simulink model "JONASBROTHERS"  (R2021b)
settings: Solver=FixedStepAuto  StartTime=0.0  StopTime=20  FixedStep=0.0001  RelTol=1e-3
model workspace (MATLAB code in the model file):
  | %% Parameters
  | m_pl = 8800;
  | r_d = 0.2323/2;
  | ig = 4;
  | J_drum = 1.0;
  | J_M = 1.5;
  | %J_M = 2.9;
  | b_hat = 15;
  | 
  | %% Speed Controller
  | t_r = 1e-3;
  | w_BW = log(9)/t_r;
  | %w_BW = 749.6586;
  | w_BWs = 0.1*w_BW;
  | %w_BWs = log(9)/0.09;
  | J_hat = m_pl*((r_d/(ig*4))^2) + J_drum*((1/ig)^2) + J_M
  | 
  | np=2;
  | p=4;
  | i_d_nl = 37.46;
  | %i_d_nl = 65.32;
  | 
  | %% Electrical Parameters
  | R_R_opt = 0.0193;
  | %R_R_opt = 0.04264;
  | R_R_hat = R_R_opt;
  | X_M_opt = 2.81;
  | %X_M_opt = 1.5829;
  | X_sig_opt = 0.0445;
  | %X_sig_opt = 0.0250;
  | omega_rN = 310.5988;
  | omega_N = 314.1593;
  | omega1 = omega_rN;
  | 
  | L_M_hat = X_M_opt/omega1;
  | L_sig_hat = X_sig_opt/omega1;
  | R_s = 0.04264;
  | %R_s = R_R_hat*1.5;
  | %psi_ref = L_M_hat * i_d_nl;
  | psi_ref = 0.8537;
  | %psi_ref = 0.70;
  | KVA = 90/0.85;
  | %V_base = (KVA*1000)/(160*1.73);
  | V_base = 400*sqrt(2)/sqrt(3);
  | alpha_fw = (2*R_R_hat)/L_sig_hat;
  | Ts = 0.0001;
  | I_max = 185;
  | 
  | kps = 2*J_hat*w_BWs/(3*np^2*psi_ref); % notes psi_R_hat is psi_ref
  | kis = w_BWs^2*2*J_hat/(3*np^2*psi_ref); % notes
  | Ba = 2*J_hat/(3*np^2*psi_ref)*(w_BWs-b_hat/J_hat); % notes
  | 
  | kp = w_BW*L_sig_hat;
  | ki = w_BW^2*L_sig_hat;
  | Ra = w_BW*L_sig_hat - (R_R_hat + R_s);
  | R = R_R_hat + R_s;
  | %% Noise
  | sigma_w = 0.5;
  | beta = 10000;
undefined symbols (not defined in the file or in its folder): j, magnitude
libraries: fl_lib x22, nesl_utility x9, CustomComponents_lib x6, simulink x6, slpidlib x2, sdl_lib x1, SignalEditorBlockLib x1
(part 1 of 2)
settings Model: Creator=Jakob  LastModifiedBy=Jakob
settings DebuggingCC: UnconnectedInputMsg=none  UnconnectedOutputMsg=none  UnconnectedLineMsg=none
settings RTWCC: DLArmComputeVersion=20.02.1

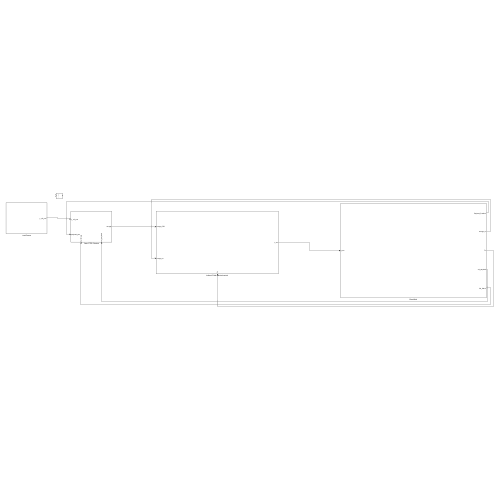
[thumbnail: Simulink's stored preview of the top-level diagram]
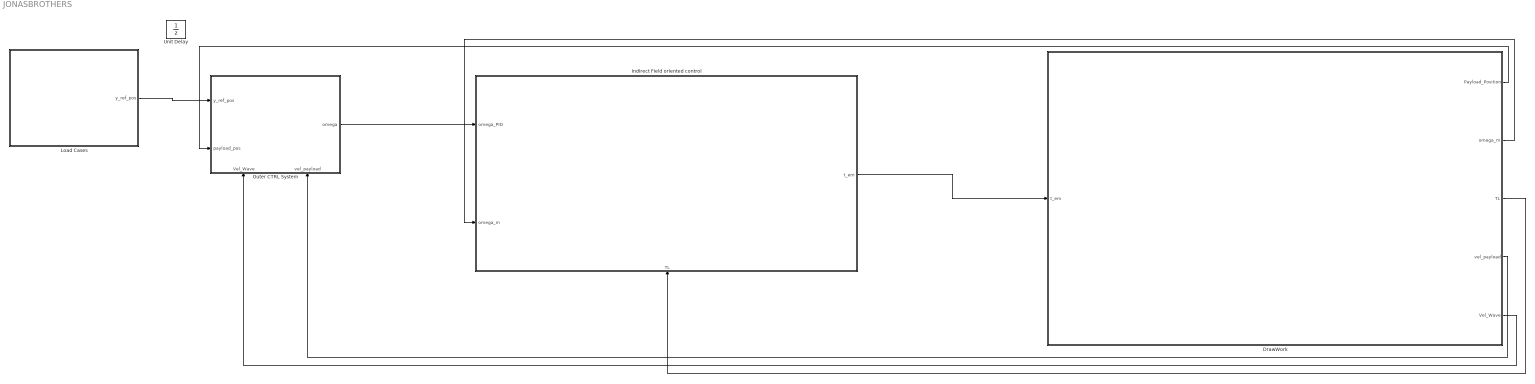
== system JONASBROTHERS ==
  DrawWork : Subsystem
  Indirect Field oriented control : Subsystem
      settings: PortSchema="{\"entries\":[{\"content\":{\"sides\":[{\"content\":{\"connectorIds\":[\"In1\",\"In2\"]},\"type\":\"ConnectorPlacement.EquallySpacedRectSide\",\"uuid\":\"3558566d-3896-4be7-a448-342d07425086\"},{\"content\":{\"connectorIds\":[\"Out1\"],\"side\":\"RIGHT\"},\"type\":\"ConnectorPlacement.EquallySpacedRectSide\",\"uuid\":\"82264b61-0ebe-4d2c-998d-795058aae34e\"},{\"content\":{\"connectorIds\":[],\"side\":\"TOP\"},\"type\":\"ConnectorPlacement.EquallySpacedRectSide\",\"uuid\":\"470bd7e5-a451-470c-b822-89589bfb916a\"},{\"content\":{\"connectorIds\":[\"In3\"],\"side\":\"BOTTOM\"},\"type\":\"ConnectorPlacement.EquallySpacedRectSide\",\"uuid\":\"a5dc14f8-1aa2-4f6b-8a94-10f64ecc4440\"}]},\"type\":\"ConnectorPlacement.EquallySpacedConnector\",\"uuid\":\"fc603cd1-8d61-44a9-91b8-960bbff8932a\"}],\"packageUris\":[\"http://schema.mathworks.com/mf0/Connector/R2020b\"],\"version\":\"1.0\"}"
  Load Cases : Subsystem
  Outer CTRL System : Subsystem
      settings: PortSchema="{\"entries\":[{\"content\":{\"sides\":[{\"content\":{\"connectorIds\":[\"In1\",\"In2\"]},\"type\":\"ConnectorPlacement.EquallySpacedRectSide\",\"uuid\":\"1b9d5986-b048-41c2-8e20-8e14a10e87ac\"},{\"content\":{\"connectorIds\":[\"Out1\"],\"side\":\"RIGHT\"},\"type\":\"ConnectorPlacement.EquallySpacedRectSide\",\"uuid\":\"6d417e58-246f-4168-97e0-db5100f5a916\"},{\"content\":{\"connectorIds\":[],\"side\":\"TOP\"},\"type\":\"ConnectorPlacement.EquallySpacedRectSide\",\"uuid\":\"d5ccf72e-5ab0-4bd7-afc9-f09220873e53\"},{\"content\":{\"connectorIds\":[\"In3\",\"In4\"],\"side\":\"BOTTOM\"},\"type\":\"ConnectorPlacement.EquallySpacedRectSide\",\"uuid\":\"d857e7ff-cab5-40fc-8d38-72d8a9d59103\"}]},\"type\":\"ConnectorPlacement.EquallySpacedConnector\",\"uuid\":\"d6c41efc-b86a-43cb-98a1-4acad2c3d840\"}],\"packageUris\":[\"http://schema.mathworks.com/mf0/Connector/R2020b\"],\"version\":\"1.0\"}"
  Unit Delay : UnitDelay  SampleTime=-1  HasFrameUpgradeWarning=on
  wires:
  DrawWork/1(Payload_Position) -> Outer CTRL System/2(payload_pos)
  DrawWork/2(omega_m) -> Indirect Field oriented control/2(omega_m)
  DrawWork/3(TL) -> Indirect Field oriented control/3(TL)
  Outer CTRL System/1(omega) -> Indirect Field oriented control/1(omega_PID)
  Indirect Field oriented control/1(t_em) -> DrawWork/1(t_em)
  DrawWork/5(Vel_Wave) -> Outer CTRL System/3(Vel_Wave)
  Load Cases/1(y_ref_pos) -> Outer CTRL System/1(y_ref_pos)
  DrawWork/4(vel_payload) -> Outer CTRL System/4(vel_payload)

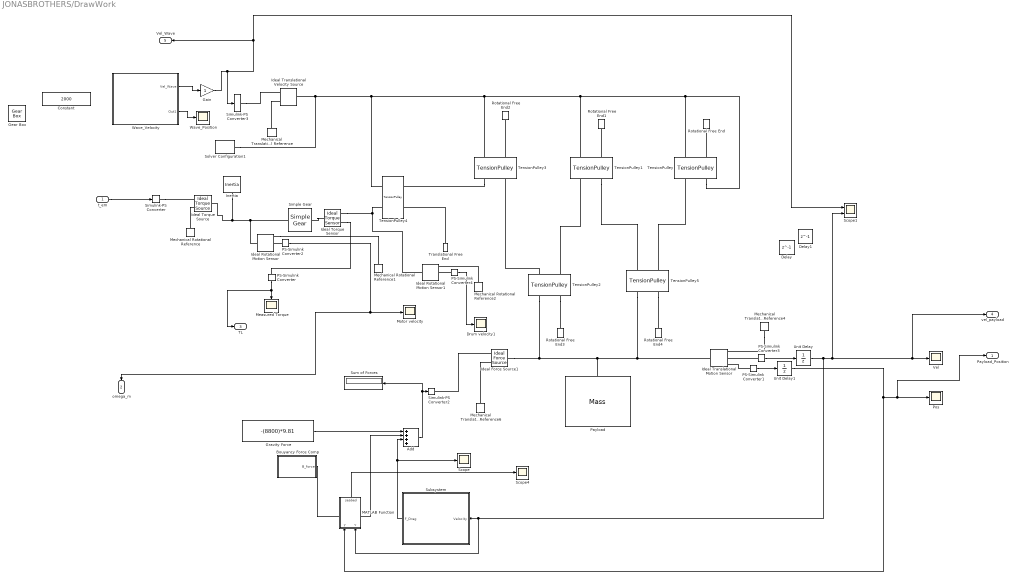
== system JONASBROTHERS/DrawWork ==
  t_em : Inport
  Add : Sum  Inputs=++++
  Bouyancy Force Comp : Subsystem
  Constant : Constant  Value=2000
  Delay : Delay  DelayLength=1  InitialCondition=75
  Delay1 : Delay  DelayLength=1  InitialCondition=0
  Drum velocity1 : Scope
  Gain : Gain
  Gear Box : fl_lib/Mechanical/Mechanisms/Gear Box  ratio=1  t_in_specify=off  t_in_priority=None  t_in=0 N*m  t_in_nominal_specify=off  t_in_nominal_unit=N*m  t_in_nominal_value=1  t_out_specify=off  t_out_priority=None  t_out=0 N*m  t_out_nominal_specify=off  t_out_nominal_unit=N*m  t_out_nominal_value=1
      settings: SourceProductBaseCode=PW,SS,VE
  Gravity Force : Constant  Value=-(8800)*9.81
  Ideal Force Source1 : fl_lib/Mechanical/Mechanical Sources/Ideal Force Source
      settings: SourceProductBaseCode=PW,SS,VE
  Ideal Rotational Motion Sensor : fl_lib/Mechanical/Mechanical Sensors/Ideal Rotational Motion Sensor  wrap_angle=simscape.enum.onoff.off  offset=0 rad
      settings: SourceProductBaseCode=PW,SS,VE
  Ideal Rotational Motion Sensor1 : fl_lib/Mechanical/Mechanical Sensors/Ideal Rotational Motion Sensor  wrap_angle=simscape.enum.onoff.off  offset=0 rad
      settings: SourceProductBaseCode=PW,SS,VE
  Ideal Torque Sensor : fl_lib/Mechanical/Mechanical Sensors/Ideal Torque Sensor
      settings: SourceProductBaseCode=PW,SS,VE
  Ideal Torque Source : fl_lib/Mechanical/Mechanical Sources/Ideal Torque Source
      settings: SourceProductBaseCode=PW,SS,VE
  Ideal Translational Motion Sensor : fl_lib/Mechanical/Mechanical Sensors/Ideal Translational Motion Sensor  offset=75 m
      settings: SourceProductBaseCode=PW,SS,VE
  Ideal Translational Velocity Source : fl_lib/Mechanical/Mechanical Sources/Ideal Translational Velocity Source
      settings: SourceProductBaseCode=PW,SS,VE
  Inertia : fl_lib/Mechanical/Rotational Elements/Inertia  inertia=1.5 kg*m^2  num_ports=foundation.enum.numPorts2.one  w_specify=off  w_priority=High  w=0 rad/s  w_nominal_specify=off  w_nominal_unit=rad/s  w_nominal_value=1  t_specify=off  t_priority=None  t=0 N*m  t_nominal_specify=off  t_nominal_unit=N*m  t_nominal_value=1
      settings: SourceProductBaseCode=PW,SS,VE
  MATLAB Function : MATLAB Function  TreatAsAtomicUnit=on
  Measured Torque : Scope
  Mechanical Rotational Reference : fl_lib/Mechanical/Rotational Elements/Mechanical Rotational Reference
      settings: SourceProductBaseCode=PW,SS,VE
  Mechanical Rotational Reference1 : fl_lib/Mechanical/Rotational Elements/Mechanical Rotational Reference
      settings: SourceProductBaseCode=PW,SS,VE
  Mechanical Rotational Reference2 : fl_lib/Mechanical/Rotational Elements/Mechanical Rotational Reference
      settings: SourceProductBaseCode=PW,SS,VE
  Mechanical Translational Reference : fl_lib/Mechanical/Translational Elements/Mechanical Translational Reference
      settings: SourceProductBaseCode=PW,SS,VE
  Mechanical Translational Reference4 : fl_lib/Mechanical/Translational Elements/Mechanical Translational Reference
      settings: SourceProductBaseCode=PW,SS,VE
  Mechanical Translational Reference6 : fl_lib/Mechanical/Translational Elements/Mechanical Translational Reference
      settings: SourceProductBaseCode=PW,SS,VE
  Motor velocity : Scope
  PS-Simulink Converter{,1..4} (5 alike) : nesl_utility/PS-Simulink Converter  PhysicalDomain=network_engine_domain  SubClassName=ps_output  LeftPortType=input  RightPortType=output  PseudoPeriodic=off  Frequencies=[]  VectorFormat=inherit  Unit=inherit  AffineConversion=off
      settings: SourceProductBaseCode=SS,PW,VE
  Payload : fl_lib/Mechanical/Translational Elements/Mass  mass=8800 kg  num_ports=foundation.enum.numPorts2.one  v_specify=off  v_priority=High  v=0 m/s  v_nominal_specify=off  v_nominal_unit=m/s  v_nominal_value=1  f_specify=off  f_priority=None  f=0 N  f_nominal_specify=off  f_nominal_unit=N  f_nominal_value=1
      settings: SourceProductBaseCode=PW,SS,VE
  Pos : Scope
  Rotational Free End{,1..4} (5 alike) : fl_lib/Mechanical/Rotational Elements/Rotational Free End  w_specify=off  w_priority=None  w=0 rad/s  w_nominal_specify=off  w_nominal_unit=rad/s  w_nominal_value=1
      settings: SourceProductBaseCode=PW,SS,VE
  Scope : Scope
  Scope1 : Scope  NumInputPorts=2
  Scope4 : Scope
  Simple Gear : sdl_lib/Gears/Simple Gear  ratio=4  rotation_direction=sdl.enum.shaftOutputDirection.same  friction_model=sdl.enum.gear_efficiencies_load.off  T_noload=0.1 N*m  T_nom=5 N*m  efficiency_nom=0.8  efficiency=0.8  temperature_TLU=[280, 300, 320] K  load_TLU=[1, 5, 10] N*m  efficiency_TLU=[.95, .9, .85]  efficiency_TLU2=[.85, .8, .75; .95, .9, .85; .85, .8, .7]  w_thr=0.01 rad/s  pwr_thr=0.001 W  backlash_model=sdl.enum.backlashModel.Off  backlash_distance=1e-3 mm  x0=0 mm  r_base=0.1 m  hardstop_model=simscape.enum.hardstop.smooth  transition=1e-4 mm  backlash_stiffness=1e7 N/m  backlash_damping=1e6 N*s/m  e=0  v_tol=0.001 m/s  mu_visc=[0, 0] N*m*s/rad  enable_faults=simscape.enum.onoff.off  efficiency_fault=0.05  external_fault=simscape.enum.onoff.off  temporal_fault=simscape.enum.onoff.off  fault_time=5 s  fault_angles=pi / 12 rad  report_fault=simscape.enum.assert.action.none  thermal_mass=50 J/K  temperature_specify=off  temperature_priority=High  temperature=300 K  temperature_nominal_specify=off  temperature_nominal_unit=K  temperature_nominal_value=1  x_backlash_specify=off  x_backlash_priority=None  x_backlash=0 mm  x_backlash_nominal_specify=off  x_backlash_nominal_unit=mm  x_backlash_nominal_value=1  f_hardstop_specify=off  f_hardstop_priority=None  f_hardstop=0 N  f_hardstop_nominal_specify=off  f_hardstop_nominal_unit=N  f_hardstop_nominal_value=1  v_backlash_specify=off  v_backlash_priority=None  v_backlash=0 m/s  v_backlash_nominal_specify=off  v_backlash_nominal_unit=m/s  v_backlash_nominal_value=1
  Simulink-PS Converter : nesl_utility/Simulink-PS Converter  PhysicalDomain=network_engine_domain  SubClassName=ps_input  LeftPortType=input  RightPortType=output  PseudoPeriodic=off  Frequencies=[]  NoiseDistribution=none  NoiseParameters=[]  Unit=N*m  AffineConversion=off  FilteringAndDerivatives=provide  SimscapeFilterOrder=1  InputFilterTimeConstant=0.001  UdotUserProvided=0
      settings: SourceProductBaseCode=SS,PW,VE
  Simulink-PS Converter2 : nesl_utility/Simulink-PS Converter  PhysicalDomain=network_engine_domain  SubClassName=ps_input  LeftPortType=input  RightPortType=output  PseudoPeriodic=off  Frequencies=[]  NoiseDistribution=none  NoiseParameters=[]  Unit=N  AffineConversion=off  FilteringAndDerivatives=provide  SimscapeFilterOrder=1  InputFilterTimeConstant=0.001  UdotUserProvided=0
      settings: SourceProductBaseCode=SS,PW,VE
  Simulink-PS Converter3 : nesl_utility/Simulink-PS Converter  PhysicalDomain=network_engine_domain  SubClassName=ps_input  LeftPortType=input  RightPortType=output  PseudoPeriodic=off  Frequencies=[]  NoiseDistribution=none  NoiseParameters=[]  Unit=m/s  AffineConversion=off  FilteringAndDerivatives=filter  SimscapeFilterOrder=1  InputFilterTimeConstant=0.001  UdotUserProvided=0
      settings: SourceProductBaseCode=SS,PW,VE
  Solver Configuration1 : nesl_utility/Solver Configuration  PhysicalDomain=network_engine_domain  SubClassName=solver  LeftPortType=input  RightPortType=generic  Tones=[]  Harmonics=[]  SimulateNoise=off  Profile=off  UseLocalSampling=off  EnableSwitchedLinearOptims=on  FrequencyDomain=off  UseCCode=off  RelTol=0.001  AbsTol=0.001  MinStep=1e-09  ToWorkspace=off  RevertToSquareIcSolve=off  NumHomotopyIterations=100  PhasorMode=off  PhasorModeNumHarmonics=1  IndexReductionMethod=DerivativeReplacement  DoDC=off  ResidualTolerance=1e-06  UseLocalSolver=off  LocalSolverChoice=NE_BACKWARD_EULER_ADVANCER  LocalSolverSampleTime=0.001  DoFixedCost=off  MaxNonlinIter=3  MaxModeIter=2  ComputeImpulses=off  ImpulseIterations=2  LinearAlgebra=auto  LinearAlgebraNumThread=0  EquationFormulation=NE_TIME_EF  DelaysMemoryBudget=1024  AutomaticFiltering=on  FilteringTimeConstant=0.001  PartitionStorageMethod=AS_NEEDED  PartitionMemoryBudget=1024  PartitionMethod=ROBUST
      settings: SourceProductBaseCode=SS,PW,VE
  Subsystem : Subsystem
  Sum of Forces : Display
  TensionPulley{,1..3,5} (5 alike) : CustomComponents_lib/TensionPulley  radius=0.01 m  b_damp=0 N*m*s/rad  inertia=0.001 kg*m^2  mass=0.1 kg  mu_s=1  f_A_specify=off  f_A_priority=None  f_A=0 N  f_A_nominal_specify=off  f_A_nominal_unit=N  f_A_nominal_value=1  f_B_specify=off  f_B_priority=None  f_B=0 N  f_B_nominal_specify=off  f_B_nominal_unit=N  f_B_nominal_value=1  f_C_specify=off  f_C_priority=None  f_C=0 N  f_C_nominal_specify=off  f_C_nominal_unit=N  f_C_nominal_value=1  tau_specify=off  tau_priority=None  tau=0 N*m  tau_nominal_specify=off  tau_nominal_unit=N*m  tau_nominal_value=1  w_specify=off  w_priority=None  w=0 rad/s  w_nominal_specify=off  w_nominal_unit=rad/s  w_nominal_value=1  v_specify=off  v_priority=None  v=0 m/s  v_nominal_specify=off  v_nominal_unit=m/s  v_nominal_value=1
      settings: InternalSimscapePortConfiguration="{\"Bottom\":[],\"Left\":[{\"id\":\"C\",\"label\":\"C\",\"type\":\"foundation.mechanical.translational.translational\"},{\"id\":\"S\",\"label\":\"S\",\"type\":\"foundation.mechanical.rotational.rotational\"}],\"Right\":[{\"id\":\"A\",\"label\":\"A\",\"type\":\"foundation.mechanical.translational.translational\"},{\"id\":\"B\",\"label\":\"B\",\"type\":\"foundation.mechanical.translational.translational\"}],\"Top\":[]}"
  TensionPulley4 : CustomComponents_lib/TensionPulley  radius=0.2323/2 m  b_damp=0.001 N*m*s/rad  inertia=1 kg*m^2  mass=1 kg  mu_s=1  f_A_specify=off  f_A_priority=None  f_A=0 N  f_A_nominal_specify=off  f_A_nominal_unit=N  f_A_nominal_value=1  f_B_specify=off  f_B_priority=None  f_B=0 N  f_B_nominal_specify=off  f_B_nominal_unit=N  f_B_nominal_value=1  f_C_specify=off  f_C_priority=None  f_C=0 N  f_C_nominal_specify=off  f_C_nominal_unit=N  f_C_nominal_value=1  tau_specify=off  tau_priority=None  tau=2000 N*m  tau_nominal_specify=off  tau_nominal_unit=N*m  tau_nominal_value=1  w_specify=off  w_priority=High  w=0 rad/s  w_nominal_specify=off  w_nominal_unit=rad/s  w_nominal_value=1  v_specify=off  v_priority=None  v=0 m/s  v_nominal_specify=off  v_nominal_unit=m/s  v_nominal_value=1
      settings: InternalSimscapePortConfiguration="{\"Bottom\":[],\"Left\":[{\"id\":\"C\",\"label\":\"C\",\"type\":\"foundation.mechanical.translational.translational\"},{\"id\":\"S\",\"label\":\"S\",\"type\":\"foundation.mechanical.rotational.rotational\"}],\"Right\":[{\"id\":\"A\",\"label\":\"A\",\"type\":\"foundation.mechanical.translational.translational\"},{\"id\":\"B\",\"label\":\"B\",\"type\":\"foundation.mechanical.translational.translational\"}],\"Top\":[]}"
  Translational Free End : fl_lib/Mechanical/Translational Elements/Translational Free End  v_specify=off  v_priority=None  v=0 m/s  v_nominal_specify=off  v_nominal_unit=m/s  v_nominal_value=1
      settings: SourceProductBaseCode=PW,SS,VE  InternalSimscapePortConfiguration="{\"Bottom\":[],\"Left\":[{\"id\":\"V\",\"label\":\"\",\"type\":\"foundation.mechanical.translational.translational\"}],\"Right\":[],\"Top\":[]}"
  Unit Delay : UnitDelay  SampleTime=-1  HasFrameUpgradeWarning=on
  Unit Delay1 : UnitDelay  InitialCondition=75  SampleTime=-1  HasFrameUpgradeWarning=on
  Vel : Scope
  Wave_Position : Scope
  Wave_Velocity : Subsystem
  Payload_Position : Outport
  omega_m : Outport  Port=2
  TL : Outport  Port=3
  vel_payload : Outport  Port=4
  Vel_Wave : Outport  Port=5
  wires:
  Subsystem/1(F_Drag) -> Scope/1, Add/3
  Bouyancy Force Comp/1(B_force) -> Add/2
  Wave_Velocity/1(Vel_Wave) -> Gain/1
  Gravity Force/1 -> Add/1
  Add/1 -> Sum of Forces/1, Simulink-PS Converter2/1
  PS-Simulink Converter/1 -> TL/1, Measured Torque/1
  MATLAB Function/1(seabed) -> Scope4/1
  PS-Simulink Converter3/1 -> Unit Delay/1
  PS-Simulink Converter1/1 -> Unit Delay1/1
  Unit Delay/1 -> MATLAB Function/2(v), Subsystem/1(Velocity), vel_payload/1, Vel/1, Scope1/2
  Unit Delay1/1 -> Pos/1, Payload_Position/1, MATLAB Function/1(y)
  t_em/1 -> Simulink-PS Converter/1
  Wave_Velocity/2(Out1) -> Wave_Position/1
  Gain/1 -> Scope1/1, Vel_Wave/1, Simulink-PS Converter3/1
  PS-Simulink Converter4/1 -> Drum velocity1/1
  PS-Simulink Converter2/1 -> Motor velocity/1, omega_m/1
  connections:
  Ideal Force Source1/LConn1 -- TensionPulley2/LConn1 -- TensionPulley5/LConn1 -- Ideal Translational Motion Sensor/LConn1 -- Payload/LConn1
  Simulink-PS Converter/RConn1 -- Ideal Torque Source/RConn1
  Ideal Force Source1/RConn1 -- Simulink-PS Converter2/RConn1
  TensionPulley/LConn2 -- Rotational Free End/LConn1
  Simulink-PS Converter3/RConn1 -- Ideal Translational Velocity Source/RConn1
  PS-Simulink Converter1/LConn1 -- Ideal Translational Motion Sensor/RConn3
  Mechanical Rotational Reference/LConn1 -- Ideal Torque Source/RConn2
  Ideal Force Source1/RConn2 -- Mechanical Translational Reference6/LConn1
  TensionPulley5/LConn2 -- Rotational Free End4/LConn1
  PS-Simulink Converter3/LConn1 -- Ideal Translational Motion Sensor/RConn2
  Mechanical Translational Reference4/LConn1 -- Ideal Translational Motion Sensor/RConn1
  TensionPulley1/LConn2 -- Rotational Free End1/LConn1
  TensionPulley3/LConn2 -- Rotational Free End2/LConn1
  TensionPulley2/LConn2 -- Rotational Free End3/LConn1
  TensionPulley/RConn2 -- TensionPulley4/LConn1 -- Solver Configuration1/RConn1 -- Ideal Translational Velocity Source/LConn1 -- TensionPulley3/LConn1 -- TensionPulley1/LConn1 -- TensionPulley/LConn1
  TensionPulley2/RConn1 -- TensionPulley3/RConn2
  TensionPulley2/RConn2 -- TensionPulley1/RConn1
  TensionPulley1/RConn2 -- TensionPulley5/RConn1
  TensionPulley5/RConn2 -- TensionPulley/RConn1
  Ideal Rotational Motion Sensor/RConn1 -- Mechanical Rotational Reference1/LConn1
  PS-Simulink Converter2/LConn1 -- Ideal Rotational Motion Sensor/RConn2
  Inertia/LConn1 -- Ideal Torque Source/LConn1 -- Ideal Rotational Motion Sensor/LConn1 -- Simple Gear/LConn1
  Ideal Torque Sensor/LConn1 -- Simple Gear/RConn1
  Ideal Torque Sensor/RConn1 -- TensionPulley4/LConn2 -- Ideal Rotational Motion Sensor1/LConn1
  Ideal Torque Sensor/RConn2 -- PS-Simulink Converter/LConn1
  Mechanical Rotational Reference2/LConn1 -- Ideal Rotational Motion Sensor1/RConn1
  PS-Simulink Converter4/LConn1 -- Ideal Rotational Motion Sensor1/RConn2
  Translational Free End/LConn1 -- TensionPulley4/RConn2
  TensionPulley3/RConn1 -- TensionPulley4/RConn1
  Ideal Translational Velocity Source/RConn2 -- Mechanical Translational Reference/LConn1

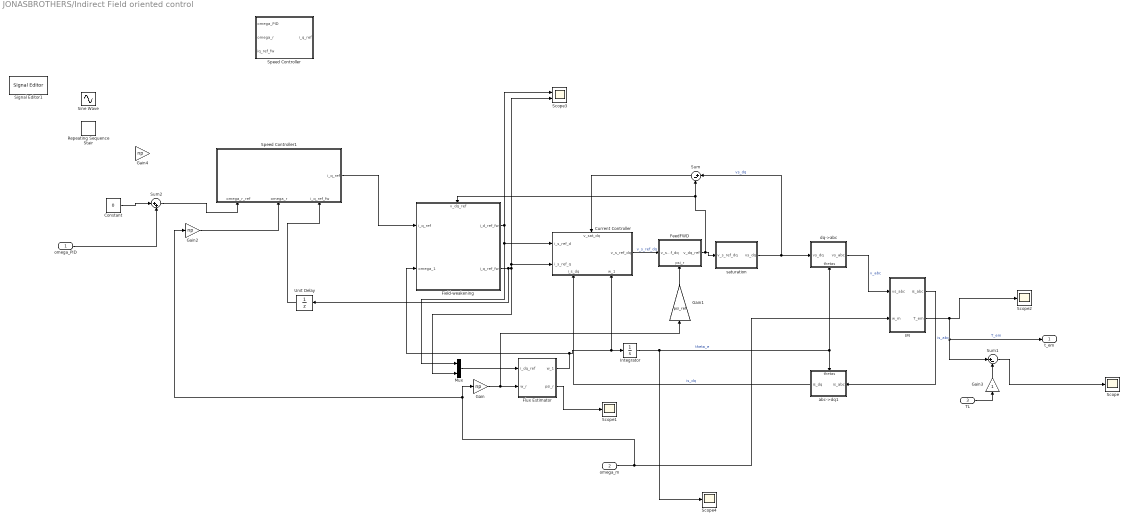
== system JONASBROTHERS/Indirect Field oriented control ==
  omega_PID : Inport
  omega_m : Inport  Port=2
  TL : Inport  Port=3
  Constant : Constant  Value=0
  Current Controller : Subsystem
      settings: PortSchema="{\"entries\":[{\"content\":{\"sides\":[{\"content\":{\"connectorIds\":[\"In1\",\"In2\"]},\"type\":\"ConnectorPlacement.EquallySpacedRectSide\",\"uuid\":\"97c548b6-6990-4323-a853-1e64e742285c\"},{\"content\":{\"connectorIds\":[\"Out1\"],\"side\":\"RIGHT\"},\"type\":\"ConnectorPlacement.EquallySpacedRectSide\",\"uuid\":\"cacb7644-0a67-4de4-9bb2-887734fe331a\"},{\"content\":{\"connectorIds\":[\"In3\"],\"side\":\"TOP\"},\"type\":\"ConnectorPlacement.EquallySpacedRectSide\",\"uuid\":\"a20c1423-7334-426c-a525-8bdb26886bc3\"},{\"content\":{\"connectorIds\":[\"In4\",\"In5\"],\"side\":\"BOTTOM\"},\"type\":\"ConnectorPlacement.EquallySpacedRectSide\",\"uuid\":\"b9821709-22a3-4c1b-ad46-11760bdb190f\"}]},\"type\":\"ConnectorPlacement.EquallySpacedConnector\",\"uuid\":\"74caaff1-86aa-4f34-8e3a-31d84a5552f1\"}],\"packageUris\":[\"http://schema.mathworks.com/mf0/Connector/R2020b\"],\"version\":\"1.0\"}"
  FeedFWD : Subsystem
      settings: AttributesFormatString=%<MinAlgLoopOccurrences>  PortSchema="{\"entries\":[{\"content\":{\"sides\":[{\"content\":{\"connectorIds\":[\"In1\"]},\"type\":\"ConnectorPlacement.EquallySpacedRectSide\",\"uuid\":\"8794a64f-49ba-4da5-9b58-fd7208420cfd\"},{\"content\":{\"connectorIds\":[\"Out1\"],\"side\":\"RIGHT\"},\"type\":\"ConnectorPlacement.EquallySpacedRectSide\",\"uuid\":\"2b8697f1-b735-400e-94f4-d8410b9cec93\"},{\"content\":{\"connectorIds\":[],\"side\":\"TOP\"},\"type\":\"ConnectorPlacement.EquallySpacedRectSide\",\"uuid\":\"d1696b87-b3df-486e-a2ce-05a5a02f4278\"},{\"content\":{\"connectorIds\":[\"In2\"],\"side\":\"BOTTOM\"},\"type\":\"ConnectorPlacement.EquallySpacedRectSide\",\"uuid\":\"350d8cbe-49a8-4b9b-a838-c09ef3fad5b2\"}]},\"type\":\"ConnectorPlacement.EquallySpacedConnector\",\"uuid\":\"fc4af688-7e97-4ab2-a125-9e3e68c4a913\"}],\"packageUris\":[\"http://schema.mathworks.com/mf0/Connector/R2020b\"],\"version\":\"1.0\"}"
  "Field-weakening " : Subsystem
      settings: PortSchema="{\"entries\":[{\"content\":{\"sides\":[{\"content\":{\"connectorIds\":[\"In1\",\"In2\"]},\"type\":\"ConnectorPlacement.EquallySpacedRectSide\",\"uuid\":\"aee381d7-3a71-45d0-966d-7af6601206c5\"},{\"content\":{\"connectorIds\":[\"Out1\",\"Out2\"],\"side\":\"RIGHT\"},\"type\":\"ConnectorPlacement.EquallySpacedRectSide\",\"uuid\":\"b4f04b7a-b16d-4ae2-8d18-1ccf45d54418\"},{\"content\":{\"connectorIds\":[\"In3\"],\"side\":\"TOP\"},\"type\":\"ConnectorPlacement.EquallySpacedRectSide\",\"uuid\":\"7d29b16c-0908-4291-9b7c-a89871d4912d\"}]},\"type\":\"ConnectorPlacement.EquallySpacedConnector\",\"uuid\":\"28c927f9-c9f1-4063-8a99-a2da52e20e9b\"}],\"packageUris\":[\"http://schema.mathworks.com/mf0/Connector/R2020b\"],\"version\":\"1.0\"}"
  Flux Estimator : Subsystem
  Gain : Gain  Gain=np
  Gain1 : Gain  Gain=psi_ref
  Gain2 : Gain  Gain=np
  Gain3 : Gain
  Gain4 : Gain  Gain=np
  IM : Subsystem  mask{R_s=R_s, L_sig=L_sig_hat, R_R=R_R_hat, n_p=2, L_M=L_M_hat}
      mask prompts: R_s "Stator resistance Rs (ohm)"; L_sig "Total leakage inductance L_sig (H)"; R_R "Rotor resistance R_R ( Ohm)"; n_p "Number of pole pairs n_p"; L_M "Magnetising inductance L_M (H)"
      mask help: dynamic model of IM
  Integrator : Integrator
  Mux : Mux  Inputs=2
  Repeating Sequence Stair : simulink/Sources/Repeating Sequence Stair  OutValues=[100 20 30 20 100 50 10 20].'  tsamp=-1  OutMin=[]  OutMax=[]  OutDataTypeStr=double  OutputDataTypeScalingMode=double  OutDataType=fixdt(0,8)  ConRadixGroup=Best Precision: Vector-wise  OutScaling=2^-12
  Scope{,1..2,4} (4 alike) : Scope
  Scope3 : Scope  NumInputPorts=2
  Signal Editor1 : SignalEditorBlockLib/Signal Editor  FileName=input.mat  ActiveScenario=Scenario  ActiveSignal=Signal  IsBus=off  OutputBusObjectStr=Bus: BusObject  SampleTime=0  Interpolate=off  ZeroCross=off  OutputAfterFinalValue=Setting to zero  Unit=inherit  PreserveSignalName=on
  Sine Wave : Sin  Amplitude=150  Frequency=0.5  SampleTime=0
  Speed Controller : Subsystem
  Speed Controller1 : Subsystem
      settings: PortSchema="{\"entries\":[{\"content\":{\"sides\":[{\"content\":{\"connectorIds\":[]},\"type\":\"ConnectorPlacement.EquallySpacedRectSide\",\"uuid\":\"97c548b6-6990-4323-a853-1e64e742285c\"},{\"content\":{\"connectorIds\":[\"Out1\"],\"side\":\"RIGHT\"},\"type\":\"ConnectorPlacement.EquallySpacedRectSide\",\"uuid\":\"cacb7644-0a67-4de4-9bb2-887734fe331a\"},{\"content\":{\"connectorIds\":[],\"side\":\"TOP\"},\"type\":\"ConnectorPlacement.EquallySpacedRectSide\",\"uuid\":\"a20c1423-7334-426c-a525-8bdb26886bc3\"},{\"content\":{\"connectorIds\":[\"In1\",\"In2\",\"In3\"],\"side\":\"BOTTOM\"},\"type\":\"ConnectorPlacement.EquallySpacedRectSide\",\"uuid\":\"b9821709-22a3-4c1b-ad46-11760bdb190f\"}]},\"type\":\"ConnectorPlacement.EquallySpacedConnector\",\"uuid\":\"74caaff1-86aa-4f34-8e3a-31d84a5552f1\"}],\"packageUris\":[\"http://schema.mathworks.com/mf0/Connector/R2020b\"],\"version\":\"1.0\"}"
  Sum : Sum  Inputs=|+-
  Sum1 : Sum  Inputs=|+-
  Sum2 : Sum  Inputs=|++
  Unit Delay : UnitDelay  InitialCondition=160*1.5  SampleTime=-1  HasFrameUpgradeWarning=on
  abc->dq1 : Subsystem
      settings: PortSchema="{\"entries\":[{\"content\":{\"sides\":[{\"content\":{\"connectorIds\":[\"In1\"]},\"type\":\"ConnectorPlacement.EquallySpacedRectSide\",\"uuid\":\"c3863cce-4a98-427c-9e63-89298f679a84\"},{\"content\":{\"connectorIds\":[\"Out1\"],\"side\":\"RIGHT\"},\"type\":\"ConnectorPlacement.EquallySpacedRectSide\",\"uuid\":\"ae3c4991-ab62-4114-9bee-e9a7348a29ce\"},{\"content\":{\"connectorIds\":[\"In2\"],\"side\":\"TOP\"},\"type\":\"ConnectorPlacement.EquallySpacedRectSide\",\"uuid\":\"fea582b6-68e0-450b-8231-0f2cf258215e\"},{\"content\":{\"connectorIds\":[],\"side\":\"BOTTOM\"},\"type\":\"ConnectorPlacement.EquallySpacedRectSide\",\"uuid\":\"4cb5cb50-d1c5-41cc-b580-d3f7a61a133b\"}]},\"type\":\"ConnectorPlacement.EquallySpacedConnector\",\"uuid\":\"936995e1-3667-4d5a-83ac-5ed23eb7cec5\"}],\"packageUris\":[\"http://schema.mathworks.com/mf0/Connector/R2020b\"],\"version\":\"1.0\"}"
  dq->abc : Subsystem
      settings: PortSchema="{\"entries\":[{\"content\":{\"sides\":[{\"content\":{\"connectorIds\":[\"In1\"]},\"type\":\"ConnectorPlacement.EquallySpacedRectSide\",\"uuid\":\"c3863cce-4a98-427c-9e63-89298f679a84\"},{\"content\":{\"connectorIds\":[\"Out1\"],\"side\":\"RIGHT\"},\"type\":\"ConnectorPlacement.EquallySpacedRectSide\",\"uuid\":\"ae3c4991-ab62-4114-9bee-e9a7348a29ce\"},{\"content\":{\"connectorIds\":[],\"side\":\"TOP\"},\"type\":\"ConnectorPlacement.EquallySpacedRectSide\",\"uuid\":\"fea582b6-68e0-450b-8231-0f2cf258215e\"},{\"content\":{\"connectorIds\":[\"In2\"],\"side\":\"BOTTOM\"},\"type\":\"ConnectorPlacement.EquallySpacedRectSide\",\"uuid\":\"09df17c4-38be-4fcd-b44b-abaf9d5b2651\"}]},\"type\":\"ConnectorPlacement.EquallySpacedConnector\",\"uuid\":\"936995e1-3667-4d5a-83ac-5ed23eb7cec5\"}],\"packageUris\":[\"http://schema.mathworks.com/mf0/Connector/R2020b\"],\"version\":\"1.0\"}"
  saturation : Subsystem
  t_em : Outport
  wires:
  Flux Estimator/1(w_1) -> Integrator/1, Current Controller/5(w_1), "Field-weakening "/2(omega_1)
  saturation/1(vs_dq) -> Sum/1, dq->abc/1(vs_dq)  "vs_dq"
  Integrator/1 -> Scope4/1, dq->abc/2(thetas), abc->dq1/2(thetas)  "theta_e"
  dq->abc/1(vs_abc) -> IM/1(vs_abc)  "v_abc"
  IM/1(is_abc) -> abc->dq1/1(is_abc)  "is_abc"
  Flux Estimator/2(psi_r) -> Scope1/1
  Sum/1 -> Current Controller/3(v_sat_dq)
  "Field-weakening "/1(i_d_ref_fw) -> Mux/1, Current Controller/1(i_s_ref_d), Scope3/1
  abc->dq1/1(is_dq) -> Current Controller/4(i_s_dq)  "is_dq"
  Gain/1 -> Gain1/1, Flux Estimator/2(w_r)
  IM/2(T_em) -> t_em/1, Sum1/1, Scope2/1  "T_em"
  Mux/1 -> Flux Estimator/1(i_dq_ref)
  TL/1 -> Gain3/1
  Gain3/1 -> Sum1/2
  "Field-weakening "/2(i_q_ref_fw) -> Unit Delay/1, Scope3/2, Current Controller/2(i_s_ref_q), Mux/2
  Sum1/1 -> Scope/1
  Gain1/1 -> FeedFWD/2(psi_r)
  Current Controller/1(v_s_ref_dq) -> FeedFWD/1(v_s_ref_dq)  "v_s_ref_dq"
  FeedFWD/1(v_dq_ref) -> "Field-weakening "/3(v_dq_ref), Sum/2, saturation/1(v_s_ref_dq)
  Gain2/1 -> Speed Controller1/2(omega_r)
  omega_m/1 -> Gain2/1, Gain/1, IM/2(w_m)
  Unit Delay/1 -> Speed Controller1/3(i_q_ref_fw)
  Constant/1 -> Sum2/1
  Sum2/1 -> Speed Controller1/1(omega_r_ref)
  omega_PID/1 -> Sum2/2
  Speed Controller1/1(i_q_ref) -> "Field-weakening "/1(i_q_ref)

== system JONASBROTHERS/Load Cases ==
  Case Selector : MATLAB Function  TreatAsAtomicUnit=on
  Constant : Constant
  Ramp : simulink/Sources/Ramp  slope=-2.5  start=0  InitialOutput=75
  Ramp1 : simulink/Sources/Ramp  slope=-1  start=0  InitialOutput=15
  Saturation : Saturate  UpperLimit=75  LowerLimit=15
  Saturation1 : Saturate  UpperLimit=15  LowerLimit=0
  Scope : Scope
  y_ref : Constant  Value=75
  y_ref_pos : Outport
  wires:
  Constant/1 -> Case Selector/4(CaseSelector)
  y_ref/1 -> Case Selector/1(Case1)
  Ramp/1 -> Saturation/1
  Saturation/1 -> Case Selector/2(Case2)
  Ramp1/1 -> Saturation1/1
  Saturation1/1 -> Case Selector/3(Case3)
  Case Selector/1(payload_ref_pos) -> Scope/1, y_ref_pos/1

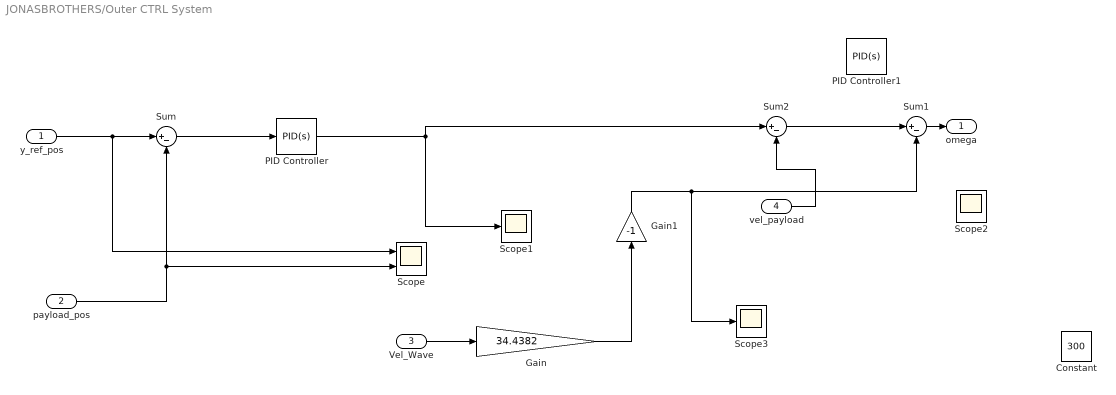
== system JONASBROTHERS/Outer CTRL System ==
  y_ref_pos : Inport
  payload_pos : Inport  Port=2
  Vel_Wave : Inport  Port=3
  vel_payload : Inport  Port=4
  Constant : Constant  Value=300
  Gain : Gain  Gain=34.4382
  Gain1 : Gain  Gain=-1
  PID Controller : slpidlib/PID Controller  Controller=PID  Form=Parallel  TimeDomain=Continuous-time  UseExternalTs=off  SampleTime=-1  IntegratorMethod=Forward Euler  FilterMethod=Forward Euler  ControllerParametersSource=internal  P=20  I=10  D=0  N=100  UseFilter=on  TunerSelectOption=Transfer Function Based (PID Tuner App)  InitialConditionSource=internal  InitialConditionForIntegrator=0  InitialConditionForFilter=0  DifferentiatorICPrevScaledInput=0  ExternalReset=none  TrackingMode=off  Kt=1  LimitOutput=off  SatLimitsSource=internal  UpperSaturationLimit=inf  LowerSaturationLimit=-inf  LinearizeAsGain=on  AntiWindupMode=none  Kb=1  POutMin=[]  POutMax=[]  IOutMin=[]  IOutMax=[]  DOutMin=[]  DOutMax=[]  NOutMin=[]  NOutMax=[]  SumOutMin=[]  SumOutMax=[]  SaturationOutMin=[]  SaturationOutMax=[]  PParamMin=[]  PParamMax=[]  IParamMin=[]  IParamMax=[]  DParamMin=[]  DParamMax=[]  NParamMin=[]  NParamMax=[]  KbParamMin=[]  KbParamMax=[]  KtParamMin=[]  KtParamMax=[]  KbOutMin=[]  KbOutMax=[]  KtOutMin=[]  KtOutMax=[]  IntegratorOutMin=[]  IntegratorOutMax=[]  FilterOutMin=[]  FilterOutMax=[]  SumI1OutMin=[]  SumI1OutMax=[]  SumI2OutMin=[]  SumI2OutMax=[]  SumI3OutMin=[]  SumI3OutMax=[]  SumI4OutMin=[]  SumI4OutMax=[]  SumDOutMin=[]  SumDOutMax=[]  DifferentiatorOutMin=[]  DifferentiatorOutMax=[]  FilterDiffOutCoefMin=[]  FilterDiffOutCoefMax=[]  ReciprocalOutMin=[]  ReciprocalOutMax=[]  SumDenOutMin=[]  SumDenOutMax=[]  SumNumOutMin=[]  SumNumOutMax=[]  DivideOutMin=[]  DivideOutMax=[]  UdiffTsProdOutMin=[]  UdiffTsProdOutMax=[]  NTsProdOutMin=[]  NTsProdOutMax=[]  UintegralTsProdOutMin=[]  UintegralTsProdOutMax=[]  UngainTsProdOutMin=[]  UngainTsProdOutMax=[]  IntegratorContinuousStateAttributes=''  IntegratorStateMustResolveToSignalObject=off  IntegratorRTWStateStorageClass=Auto  FilterContinuousStateAttributes=''  FilterStateMustResolveToSignalObject=off  FilterRTWStateStorageClass=Auto  ParallelPVariant=InternalParameters  IdealPVariant=Disabled  IVariant=InternalParameters  DVariant=InternalParameters  IntegratorVariant=Continuous  SatVariant=Disabled  AWVariant=Passthrough  PCopyVariant=Disabled  TRVariant=Disabled  FdbkBlocksVariant=Forward  IdealPFdbkVariant=Disabled  SatFdbkVariant=Disabled  DerivativeFilterVariant=ContFilter  NVariant=InternalParameters  NCopyVariant=Disabled  FilterICVariant=InternalICsFilter  IntegratorICVariant=InternalICs  ExternalResetVariant=Disabled  TRSumVariant=Passthrough  SumFdbkVariant=Disabled  SumVariant=Sum_PID  TsampFilterVariant=InternalTs  TsampNgainVariant=Passthrough  TsampIntegralVariant=Passthrough  ExternalSaturationOutDataTypeStr=Inherit: Same as second input
  PID Controller1 : slpidlib/PID Controller  Controller=PID  Form=Parallel  TimeDomain=Continuous-time  UseExternalTs=off  SampleTime=-1  IntegratorMethod=Forward Euler  FilterMethod=Forward Euler  ControllerParametersSource=internal  P=100  I=3000  D=0  N=100  UseFilter=on  TunerSelectOption=Transfer Function Based (PID Tuner App)  InitialConditionSource=internal  InitialConditionForIntegrator=0  InitialConditionForFilter=0  DifferentiatorICPrevScaledInput=0  ExternalReset=none  TrackingMode=off  Kt=1  LimitOutput=off  SatLimitsSource=internal  UpperSaturationLimit=inf  LowerSaturationLimit=-inf  LinearizeAsGain=on  AntiWindupMode=none  Kb=1  POutMin=[]  POutMax=[]  IOutMin=[]  IOutMax=[]  DOutMin=[]  DOutMax=[]  NOutMin=[]  NOutMax=[]  SumOutMin=[]  SumOutMax=[]  SaturationOutMin=[]  SaturationOutMax=[]  PParamMin=[]  PParamMax=[]  IParamMin=[]  IParamMax=[]  DParamMin=[]  DParamMax=[]  NParamMin=[]  NParamMax=[]  KbParamMin=[]  KbParamMax=[]  KtParamMin=[]  KtParamMax=[]  KbOutMin=[]  KbOutMax=[]  KtOutMin=[]  KtOutMax=[]  IntegratorOutMin=[]  IntegratorOutMax=[]  FilterOutMin=[]  FilterOutMax=[]  SumI1OutMin=[]  SumI1OutMax=[]  SumI2OutMin=[]  SumI2OutMax=[]  SumI3OutMin=[]  SumI3OutMax=[]  SumI4OutMin=[]  SumI4OutMax=[]  SumDOutMin=[]  SumDOutMax=[]  DifferentiatorOutMin=[]  DifferentiatorOutMax=[]  FilterDiffOutCoefMin=[]  FilterDiffOutCoefMax=[]  ReciprocalOutMin=[]  ReciprocalOutMax=[]  SumDenOutMin=[]  SumDenOutMax=[]  SumNumOutMin=[]  SumNumOutMax=[]  DivideOutMin=[]  DivideOutMax=[]  UdiffTsProdOutMin=[]  UdiffTsProdOutMax=[]  NTsProdOutMin=[]  NTsProdOutMax=[]  UintegralTsProdOutMin=[]  UintegralTsProdOutMax=[]  UngainTsProdOutMin=[]  UngainTsProdOutMax=[]  IntegratorContinuousStateAttributes=''  IntegratorStateMustResolveToSignalObject=off  IntegratorRTWStateStorageClass=Auto  FilterContinuousStateAttributes=''  FilterStateMustResolveToSignalObject=off  FilterRTWStateStorageClass=Auto  ParallelPVariant=InternalParameters  IdealPVariant=Disabled  IVariant=InternalParameters  DVariant=InternalParameters  IntegratorVariant=Continuous  SatVariant=Disabled  AWVariant=Passthrough  PCopyVariant=Disabled  TRVariant=Disabled  FdbkBlocksVariant=Forward  IdealPFdbkVariant=Disabled  SatFdbkVariant=Disabled  DerivativeFilterVariant=ContFilter  NVariant=InternalParameters  NCopyVariant=Disabled  FilterICVariant=InternalICsFilter  IntegratorICVariant=InternalICs  ExternalResetVariant=Disabled  TRSumVariant=Passthrough  SumFdbkVariant=Disabled  SumVariant=Sum_PID  TsampFilterVariant=InternalTs  TsampNgainVariant=Passthrough  TsampIntegralVariant=Passthrough  ExternalSaturationOutDataTypeStr=Inherit: Same as second input
  Scope : Scope  NumInputPorts=2
  Scope1 : Scope
  Scope2 : Scope
  Scope3 : Scope
  Sum : Sum  Inputs=|+-
  Sum1 : Sum  Inputs=|+-
  Sum2 : Sum  Inputs=|+-
  omega : Outport
  wires:
  payload_pos/1 -> Scope/2, Sum/2
  Sum/1 -> PID Controller/1
  y_ref_pos/1 -> Scope/1, Sum/1
  Vel_Wave/1 -> Gain/1
  Gain/1 -> Gain1/1
  Gain1/1 -> Sum1/2, Scope3/1
  PID Controller/1 -> Sum2/1, Scope1/1
  vel_payload/1 -> Sum2/2
  Sum2/1 -> Sum1/1
  Sum1/1 -> omega/1

== system JONASBROTHERS/DrawWork/Bouyancy Force Comp ==
  Constant : Constant  Value=1025
  Display : Display
  Payload Volume : Constant  Value=2
  Product : Product  Inputs=3
  gravity : Constant  Value=9.81
  B_force : Outport
  wires:
  Constant/1 -> Product/1
  Payload Volume/1 -> Product/2
  gravity/1 -> Product/3
  Product/1 -> Display/1, B_force/1

== system JONASBROTHERS/DrawWork/Subsystem ==
  Velocity : Inport
  MATLAB Function : MATLAB Function  TreatAsAtomicUnit=on
  Scope : Scope
  F_Drag : Outport
  wires:
  Velocity/1 -> MATLAB Function/1(v)
  MATLAB Function/1(F_D) -> Scope/1, F_Drag/1

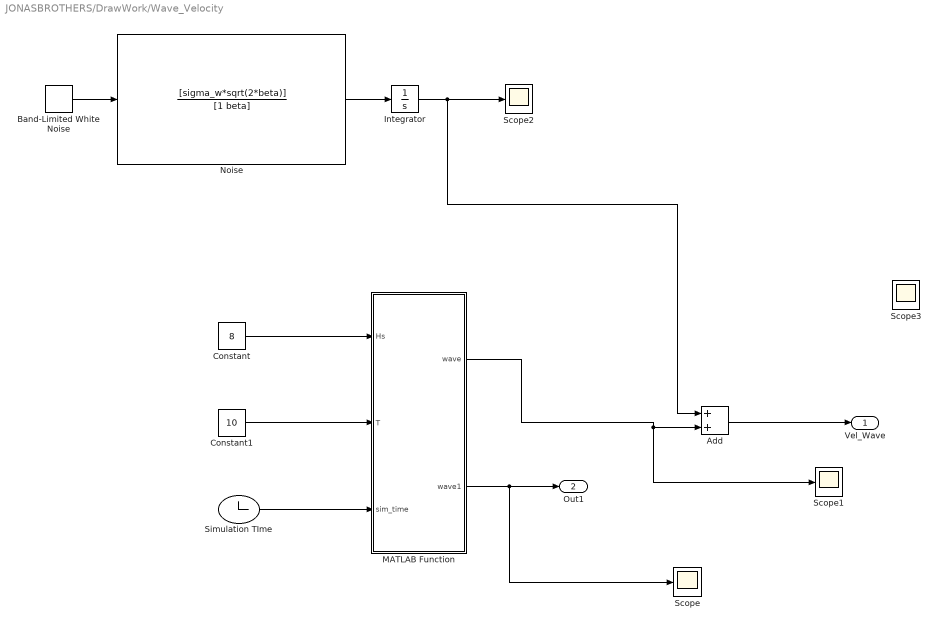
== system JONASBROTHERS/DrawWork/Wave_Velocity ==
  Add : Sum
  Band-Limited White Noise : simulink/Sources/Band-Limited White Noise  Cov=[1]  Ts=0.001  seed=[23341]
  Constant : Constant  Value=8
  Constant1 : Constant  Value=10
  Integrator : Integrator
  MATLAB Function : MATLAB Function  TreatAsAtomicUnit=on
  Noise : TransferFcn  Numerator=[sigma_w*sqrt(2*beta)]  Denominator=[1 beta]
  Scope{,1..3} (4 alike) : Scope
  Simulation TIme : Clock
      settings: Decimation=100
  Vel_Wave : Outport
  Out1 : Outport  Port=2
  wires:
  Constant/1 -> MATLAB Function/1(Hs)
  Simulation TIme/1 -> MATLAB Function/3(sim_time)
  Constant1/1 -> MATLAB Function/2(T)
  Band-Limited White Noise/1 -> Noise/1
  Noise/1 -> Integrator/1
  MATLAB Function/1(wave) -> Add/2, Scope1/1
  MATLAB Function/2(wave1) -> Scope/1, Out1/1
  Integrator/1 -> Add/1, Scope2/1
  Add/1 -> Vel_Wave/1

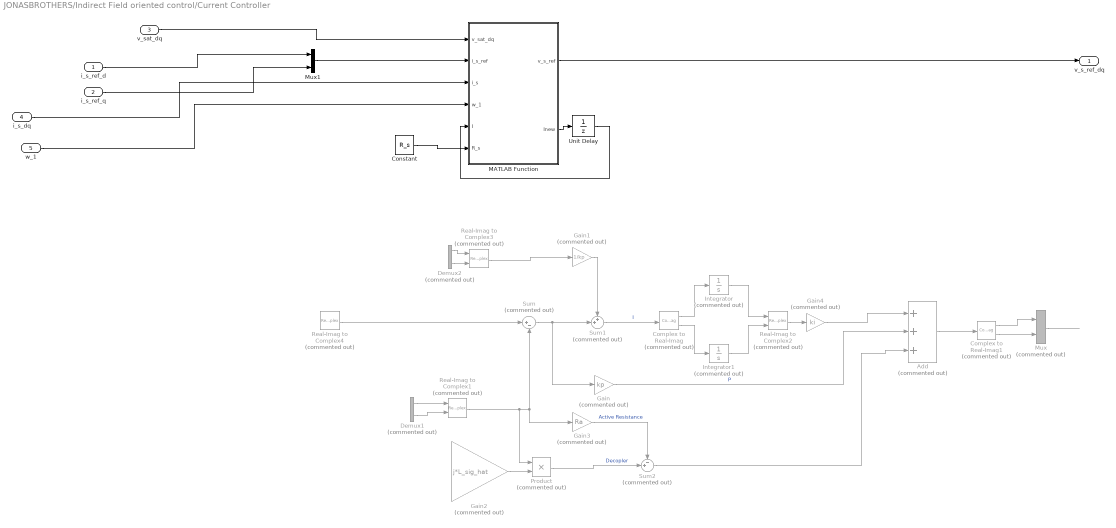
== system JONASBROTHERS/Indirect Field oriented control/Current Controller ==
  i_s_ref_d : Inport
  i_s_ref_q : Inport  Port=2
  v_sat_dq : Inport  Port=3
  i_s_dq : Inport  Port=4
  w_1 : Inport  Port=5
  Add : Sum  Commented=on  Inputs=+++
  Complex to Real-Imag : ComplexToRealImag  Commented=on
  Complex to Real-Imag1 : ComplexToRealImag  Commented=on
  Constant : Constant  Value=R_s
  Demux1 : Demux  Commented=on  Outputs=2
  Demux2 : Demux  Commented=on  Outputs=2
  Gain : Gain  Commented=on  Gain=kp
  Gain1 : Gain  Commented=on  Gain=1/kp
  Gain2 : Gain  Commented=on  Gain=j*L_sig_hat
  Gain3 : Gain  Commented=on  Gain=Ra
  Gain4 : Gain  Commented=on  Gain=ki
  Integrator : Integrator  Commented=on
  Integrator1 : Integrator  Commented=on
  MATLAB Function : MATLAB Function  TreatAsAtomicUnit=on
  Mux : Mux  Commented=on  Inputs=2
  Mux1 : Mux  Inputs=2
  Product : Product  Commented=on
  Real-Imag to Complex{1..4} (4 alike) : RealImagToComplex  Commented=on
  Sum : Sum  Commented=on  Inputs=|+-
  Sum1 : Sum  Commented=on  Inputs=++|
  Sum2 : Sum  Commented=on  Inputs=-+|
  Unit Delay : UnitDelay  SampleTime=-1  HasFrameUpgradeWarning=on
  v_s_ref_dq : Outport  PortDimensions=2
  wires:
  MATLAB Function/2(Inew) -> Unit Delay/1
  Mux1/1 -> MATLAB Function/2(i_s_ref)
  w_1/1 -> MATLAB Function/4(w_1)
  i_s_dq/1 -> MATLAB Function/3(i_s)
  Unit Delay/1 -> MATLAB Function/5(I)
  MATLAB Function/1(v_s_ref) -> v_s_ref_dq/1
  v_sat_dq/1 -> MATLAB Function/1(v_sat_dq)
  Constant/1 -> MATLAB Function/6(R_s)
  Real-Imag to Complex4/1 -> Sum/1
  Demux1/2 -> Real-Imag to Complex1/2
  Demux1/1 -> Real-Imag to Complex1/1
  Real-Imag to Complex1/1 -> Product/1, Sum/2, Gain3/1
  Sum/1 -> Gain/1, Sum1/2
  Sum1/1 -> Complex to Real-Imag/1  "I"
  Complex to Real-Imag/2 -> Integrator1/1
  Complex to Real-Imag/1 -> Integrator/1
  Integrator/1 -> Real-Imag to Complex2/1
  Integrator1/1 -> Real-Imag to Complex2/2
  Gain1/1 -> Sum1/1
  Gain2/1 -> Product/2
  ? -> Demux1/1
  ? -> Gain2/1
  Real-Imag to Complex2/1 -> Gain4/1
  Add/1 -> Complex to Real-Imag1/1
  Complex to Real-Imag1/2 -> Mux/2
  Complex to Real-Imag1/1 -> Mux/1
  Mux/1 -> ?
  Demux2/2 -> Real-Imag to Complex3/2
  Demux2/1 -> Real-Imag to Complex3/1
  ? -> Real-Imag to Complex4/1
  ? -> Real-Imag to Complex4/2
  Product/1 -> Sum2/2  "Decopler"
  Gain3/1 -> Sum2/1  "Active Resistance"
  Sum2/1 -> Add/3
  Gain4/1 -> Add/1
  Gain/1 -> Add/2  "P"
  Real-Imag to Complex3/1 -> Gain1/1
  i_s_ref_d/1 -> Mux1/1
  i_s_ref_q/1 -> Mux1/2
  ? -> Demux2/1

== system JONASBROTHERS/Indirect Field oriented control/FeedFWD ==
  v_s_ref_dq : Inport
  psi_r : Inport  Port=2
  Constant : Constant  Value=R_R_hat/L_M_hat * psi_ref
  Demux : Demux  Outputs=2
  Gain : Gain
  Mux : Mux  Inputs=2
  Sum : Sum  Inputs=-+|
  Sum1 : Sum  Inputs=|++
  v_dq_ref : Outport
  wires:
  v_s_ref_dq/1 -> Demux/1
  Mux/1 -> v_dq_ref/1
  Sum/1 -> Mux/1
  Demux/1 -> Sum/2
  Constant/1 -> Sum/1
  Demux/2 -> Sum1/1
  Sum1/1 -> Mux/2
  psi_r/1 -> Gain/1
  Gain/1 -> Sum1/2

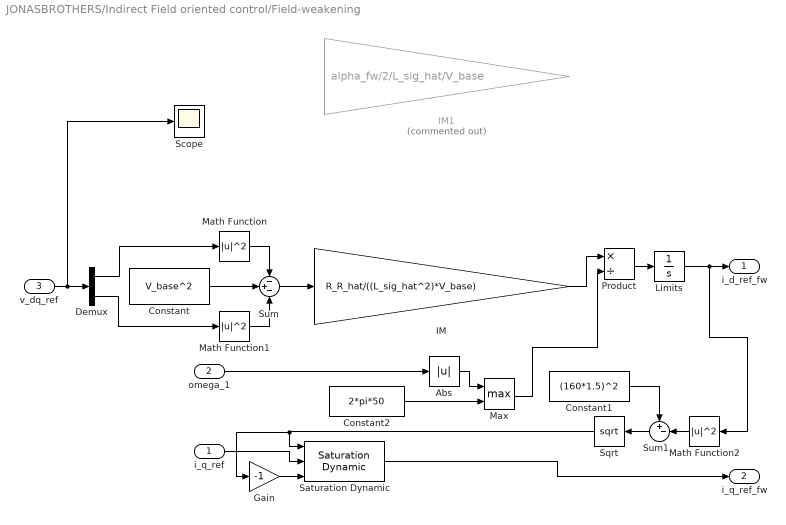
== system JONASBROTHERS/Indirect Field oriented control/Field-weakening  ==
  i_q_ref : Inport
  omega_1 : Inport  Port=2
  v_dq_ref : Inport  Port=3
  Abs : Abs
  Constant : Constant  Value=V_base^2
  Constant1 : Constant  Value=(160*1.5)^2
  Constant2 : Constant  Value=2*pi*50
  Demux : Demux  Outputs=2
  Gain : Gain  Gain=-1
  IM : Gain  Gain=R_R_hat/((L_sig_hat^2)*V_base)
  IM1 : Gain  Commented=on  Gain=alpha_fw/2/L_sig_hat/V_base
  Limits : Integrator  InitialCondition=psi_ref/L_M_hat  LimitOutput=on  UpperSaturationLimit=psi_ref/L_M_hat  LowerSaturationLimit=0.1*psi_ref/L_M_hat
  Math Function : Math  Operator=magnitude^2  SaturateOnIntegerOverflow=on
  Math Function1 : Math  Operator=magnitude^2  SaturateOnIntegerOverflow=on
  Math Function2 : Math  Operator=magnitude^2  SaturateOnIntegerOverflow=on
  Max : MinMax  Function=max  Inputs=2
  Product : Product  Inputs=*/
  Saturation Dynamic : simulink/Discontinuities/Saturation Dynamic  OutMin=[]  OutMax=[]  OutDataTypeStr=Inherit: Same as second input  OutDataType=fixdt(1, 16)  OutScaling=2^-10  DoSatur=off
  Scope : Scope
  Sqrt : Sqrt  SaturateOnIntegerOverflow=on
  Sum : Sum  Inputs=-+-
  Sum1 : Sum  Inputs=+-|
  i_d_ref_fw : Outport
  i_q_ref_fw : Outport  Port=2
  wires:
  i_q_ref/1 -> Saturation Dynamic/2
  Constant/1 -> Sum/2
  Math Function/1 -> Sum/1
  Math Function1/1 -> Sum/3
  Sum/1 -> IM/1
  IM/1 -> Product/1
  omega_1/1 -> Abs/1
  Abs/1 -> Max/1
  Max/1 -> Product/2
  Product/1 -> Limits/1
  Limits/1 -> i_d_ref_fw/1, Math Function2/1
  Math Function2/1 -> Sum1/2
  Constant1/1 -> Sum1/1
  Sum1/1 -> Sqrt/1
  Sqrt/1 -> Gain/1, Saturation Dynamic/1
  Gain/1 -> Saturation Dynamic/3
  Constant2/1 -> Max/2
  v_dq_ref/1 -> Scope/1, Demux/1
  Demux/1 -> Math Function/1
  Demux/2 -> Math Function1/1
  Saturation Dynamic/1 -> i_q_ref_fw/1

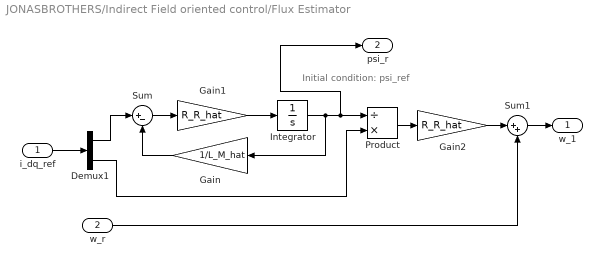
== system JONASBROTHERS/Indirect Field oriented control/Flux Estimator ==
  note: Initial condition: psi_ref
  i_dq_ref : Inport
  w_r : Inport  Port=2
  Demux1 : Demux  Outputs=2
  Gain : Gain  Gain=1/L_M_hat
  Gain1 : Gain  Gain=R_R_hat
  Gain2 : Gain  Gain=R_R_hat
  Integrator : Integrator  InitialCondition=psi_ref
  Product : Product  Inputs=/*
  Sum : Sum  Inputs=|+-
  Sum1 : Sum  Inputs=|++
  w_1 : Outport
  psi_r : Outport  Port=2
  wires:
  Product/1 -> Gain2/1
  Demux1/2 -> Product/2
  Gain1/1 -> Integrator/1
  Sum/1 -> Gain1/1
  Gain/1 -> Sum/2
  Integrator/1 -> Gain/1, psi_r/1, Product/1
  i_dq_ref/1 -> Demux1/1
  Demux1/1 -> Sum/1
  w_r/1 -> Sum1/2
  Gain2/1 -> Sum1/1
  Sum1/1 -> w_1/1

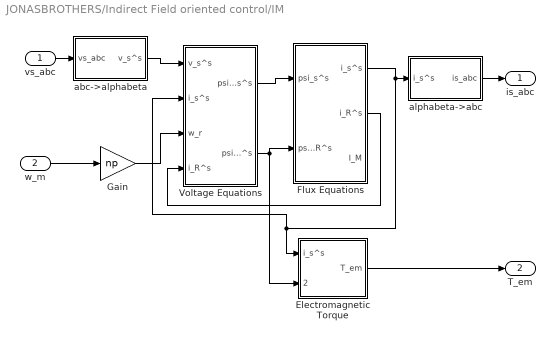
== system JONASBROTHERS/Indirect Field oriented control/IM ==
  vs_abc : Inport
  w_m : Inport  Port=2
  Electromagnetic Torque : Subsystem
  Flux Equations : Subsystem
  Gain : Gain  Gain=np  SaturateOnIntegerOverflow=on  OutDataTypeStr=Inherit: Same as input  ParamDataTypeStr=Inherit: Same as input
  Voltage Equations : Subsystem
  abc->alphabeta : Subsystem
  alphabeta->abc : Subsystem
  is_abc : Outport
  T_em : Outport  Port=2
  wires:
  Gain/1 -> Voltage Equations/3(w_r)
  alphabeta->abc/1(is_abc) -> is_abc/1
  abc->alphabeta/1(v_s^s) -> Voltage Equations/1(v_s^s)
  Voltage Equations/1(psi_s^s) -> Flux Equations/1(psi_s^s)
  Voltage Equations/2(psi_R^s) -> Flux Equations/2(psi_R^s), Electromagnetic Torque/2(psi_R^s)
  vs_abc/1 -> abc->alphabeta/1(vs_abc)
  Flux Equations/1(i_s^s) -> Electromagnetic Torque/1(i_s^s), Voltage Equations/2(i_s^s), alphabeta->abc/1(i_s^s)
  Electromagnetic Torque/1(T_em) -> T_em/1
  w_m/1 -> Gain/1
  Flux Equations/2(i_R^s) -> Voltage Equations/4(i_R^s)

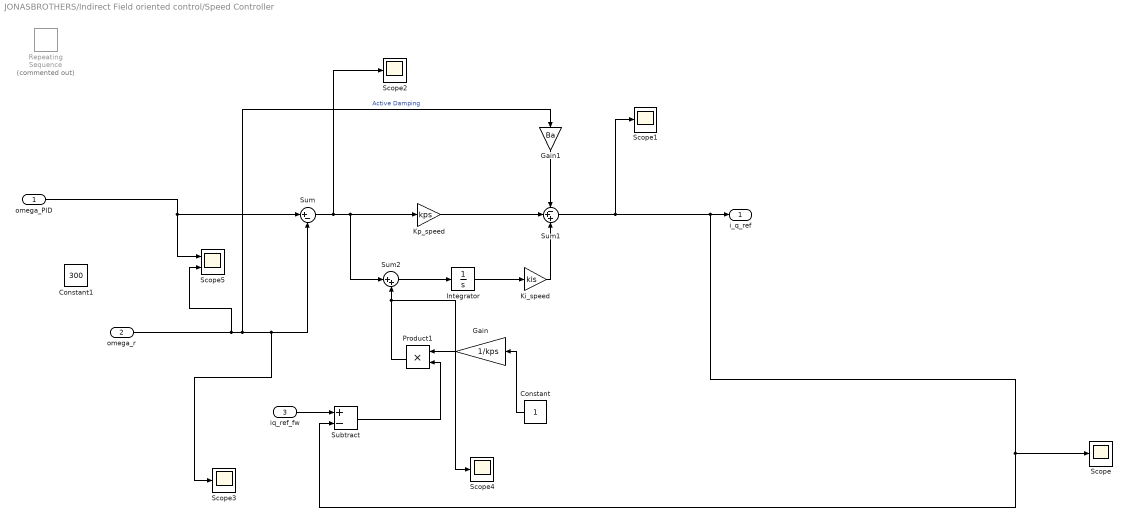
== system JONASBROTHERS/Indirect Field oriented control/Speed Controller ==
  omega_PID : Inport
  omega_r : Inport  Port=2
  iq_ref_fw : Inport  Port=3
  Constant : Constant
  Constant1 : Constant  Value=300
  Gain : Gain  Gain=1/kps
  Gain1 : Gain  Gain=Ba
  Integrator : Integrator
  Ki_speed : Gain  Gain=kis
  Kp_speed : Gain  Gain=kps
  Product1 : Product
  Repeating Sequence : simulink/Sources/Repeating Sequence  Commented=on  rep_seq_t=[0 Ts*1e3 5 5+Ts*1e3 10]*1e-3  rep_seq_y=[4.3 4.3 4.3 1 1]
  Scope{,1..4} (5 alike) : Scope
  Scope5 : Scope  NumInputPorts=2
  Subtract : Sum  Inputs=+-
  Sum : Sum  Inputs=|+-
  Sum1 : Sum  Inputs=-++
  Sum2 : Sum  Inputs=|++
  i_q_ref : Outport
  wires:
  omega_r/1 -> Scope5/2, Scope3/1, Sum/2, Gain1/1  "Active Damping"
  Sum/1 -> Scope2/1, Sum2/1, Kp_speed/1
  Kp_speed/1 -> Sum1/2
  Ki_speed/1 -> Sum1/3
  Gain1/1 -> Sum1/1
  iq_ref_fw/1 -> Subtract/1
  Gain/1 -> Product1/1
  Subtract/1 -> Product1/2
  Constant/1 -> Gain/1
  Sum1/1 -> Scope/1, Subtract/2, i_q_ref/1, Scope1/1
  Integrator/1 -> Ki_speed/1
  Sum2/1 -> Integrator/1
  Product1/1 -> Scope4/1, Sum2/2
  omega_PID/1 -> Scope5/1, Sum/1

== system JONASBROTHERS/Indirect Field oriented control/Speed Controller1 ==
  omega_r_ref : Inport
  omega_r : Inport  Port=2
  i_q_ref_fw : Inport  Port=3
  Constant : Constant  Value=np
  MATLAB Function : MATLAB Function  Commented=on  TreatAsAtomicUnit=on
  MATLAB Function1 : MATLAB Function  TreatAsAtomicUnit=on
  Scope : Scope  NumInputPorts=2
  Unit Delay : UnitDelay  SampleTime=-1  HasFrameUpgradeWarning=on
  i_q_ref : Outport  PortDimensions=1
  wires:
  MATLAB Function/2(Inew) -> ?
  ? -> MATLAB Function/2(omega_r)
  ? -> MATLAB Function/4(I)
  ? -> MATLAB Function/3(i_q_ref_fw)
  ? -> MATLAB Function/1(omega_r_ref)
  MATLAB Function1/2(Inew) -> Unit Delay/1
  Unit Delay/1 -> MATLAB Function1/4(I)
  omega_r_ref/1 -> Scope/1, MATLAB Function1/1(omega_r_ref)
  omega_r/1 -> Scope/2, MATLAB Function1/2(omega_r)
  i_q_ref_fw/1 -> MATLAB Function1/3(i_q_ref_fw)
  MATLAB Function1/1(i_q_ref) -> i_q_ref/1
  Constant/1 -> MATLAB Function1/5(np)

== system JONASBROTHERS/Indirect Field oriented control/abc->dq1 ==
  is_abc : Inport
  thetas : Inport  Port=2
  MATLAB Function : MATLAB Function  TreatAsAtomicUnit=on
  Scope : Scope
  is_dq : Outport
  wires:
  thetas/1 -> MATLAB Function/2(thetas)
  is_abc/1 -> MATLAB Function/1(is_abc)
  MATLAB Function/1(is) -> Scope/1, is_dq/1

== system JONASBROTHERS/Indirect Field oriented control/dq->abc ==
  vs_dq : Inport
  thetas : Inport  Port=2
  MATLAB Function : MATLAB Function  TreatAsAtomicUnit=on
  Scope : Scope
  vs_abc : Outport
  wires:
  vs_dq/1 -> MATLAB Function/1(vs_dq)
  thetas/1 -> MATLAB Function/2(thetas)
  MATLAB Function/1(vs_abc) -> Scope/1, vs_abc/1

== system JONASBROTHERS/Indirect Field oriented control/saturation ==
  v_s_ref_dq : Inport
  Complex to Magnitude-Angle : ComplexToMagnitudeAngle
  Complex to Real-Imag : ComplexToRealImag
  Demux1 : Demux  Outputs=2
  Magnitude-Angle to Complex : MagnitudeAngleToComplex
  Mux1 : Mux  Inputs=2
  Real-Imag to Complex : RealImagToComplex
  Saturation : Saturate  UpperLimit=400*sqrt(2)*sqrt(3)  LowerLimit=0
  vs_dq : Outport
  wires:
  Mux1/1 -> vs_dq/1
  Demux1/2 -> Real-Imag to Complex/2
  Complex to Real-Imag/1 -> Mux1/1
  Magnitude-Angle to Complex/1 -> Complex to Real-Imag/1
  Demux1/1 -> Real-Imag to Complex/1
  Real-Imag to Complex/1 -> Complex to Magnitude-Angle/1
  Complex to Real-Imag/2 -> Mux1/2
  v_s_ref_dq/1 -> Demux1/1
  Complex to Magnitude-Angle/1 -> Saturation/1
  Saturation/1 -> Magnitude-Angle to Complex/1  "sat"
  Complex to Magnitude-Angle/2 -> Magnitude-Angle to Complex/2

== system JONASBROTHERS/Indirect Field oriented control/IM/Electromagnetic Torque ==
  note: lecture 5 equation 26
  i_s^s : Inport
  psi_R^s : Inport  Port=2
  Complex to Real-Imag : ComplexToRealImag  Output=Imag
  Gain : Gain  Gain=3*np/2
  Product : Product
  conj : Math  Operator=conj  SaturateOnIntegerOverflow=on
  T_em : Outport
  wires:
  psi_R^s/1 -> conj/1
  i_s^s/1 -> Product/1
  conj/1 -> Product/2
  Product/1 -> Complex to Real-Imag/1
  Complex to Real-Imag/1 -> Gain/1
  Gain/1 -> T_em/1

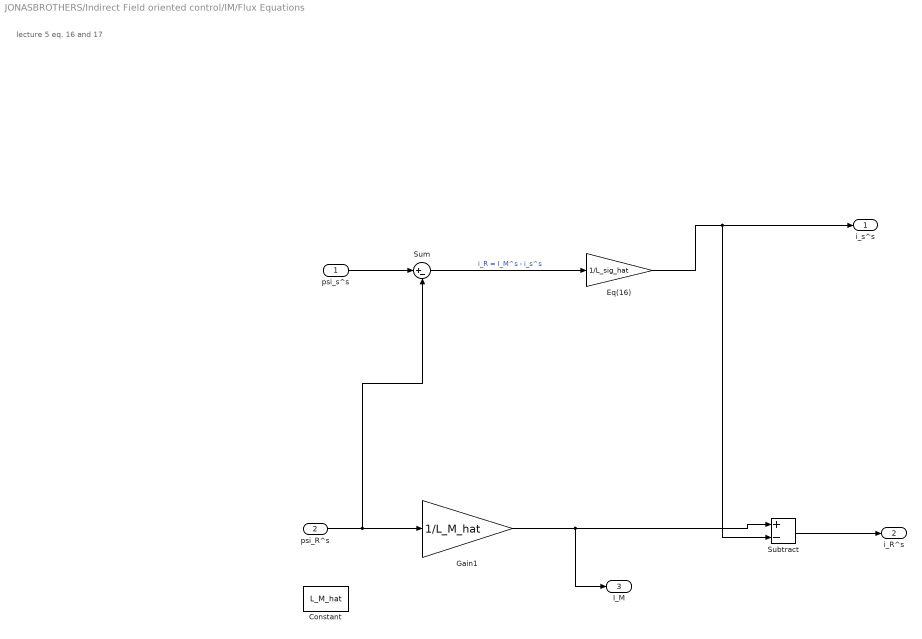
== system JONASBROTHERS/Indirect Field oriented control/IM/Flux Equations ==
  note: lecture 5 eq. 16 and 17
  psi_s^s : Inport
  psi_R^s : Inport  Port=2
  Constant : Constant  Value=L_M_hat
  Eq(16) : Gain  Gain=1/L_sig_hat
  Gain1 : Gain  Gain=1/L_M_hat
  Subtract : Sum  Inputs=+-
  Sum : Sum  Inputs=|+-
  i_s^s : Outport
  i_R^s : Outport  Port=2
  I_M : Outport  Port=3
  wires:
  psi_s^s/1 -> Sum/1
  Sum/1 -> Eq(16)/1  "i_R = I_M^s - i_s^s"
  psi_R^s/1 -> Gain1/1, Sum/2
  Subtract/1 -> i_R^s/1
  Eq(16)/1 -> Subtract/2, i_s^s/1
  Gain1/1 -> I_M/1, Subtract/1

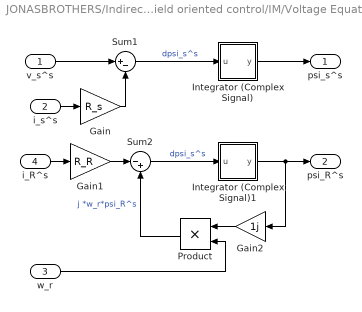
== system JONASBROTHERS/Indirect Field oriented control/IM/Voltage Equations ==
  v_s^s : Inport
  i_s^s : Inport  Port=2
  w_r : Inport  Port=3
  i_R^s : Inport  Port=4
  Gain : Gain  Gain=R_s
  Gain1 : Gain  Gain=R_R
  Gain2 : Gain  Gain=1j
  Integrator (Complex Signal) : Subsystem
      mask Display: disp('1/s');
  Integrator (Complex Signal)1 : Subsystem
      mask Display: disp('1/s');
  Product : Product  RndMeth=Zero
  Sum1 : Sum  Inputs=|+-
  Sum2 : Sum  Inputs=|-+
  psi_s^s : Outport
  psi_R^s : Outport  Port=2
  wires:
  w_r/1 -> Product/2
  Gain2/1 -> Product/1
  Integrator (Complex Signal)1/1(y) -> Gain2/1, psi_R^s/1
  Integrator (Complex Signal)/1(y) -> psi_s^s/1
  Gain/1 -> Sum1/2
  Sum1/1 -> Integrator (Complex Signal)/1(u)  "dpsi_s^s"
  i_s^s/1 -> Gain/1
  v_s^s/1 -> Sum1/1
  Product/1 -> Sum2/2  "j *w_r*psi_R^s"
  i_R^s/1 -> Gain1/1
  Gain1/1 -> Sum2/1
  Sum2/1 -> Integrator (Complex Signal)1/1(u)  "dpsi_s^s"

== system JONASBROTHERS/Indirect Field oriented control/IM/abc->alphabeta ==
  vs_abc : Inport
  Fcn : Fcn  Expr=2/3*(u(1)-0.5*u(2)-0.5*u(3))
  Fcn1 : Fcn  Expr=sqrt(3)/3*(u(2)-u(3))
  Real-Imag to Complex : RealImagToComplex
  v_s^s : Outport
  wires:
  Real-Imag to Complex/1 -> v_s^s/1
  Fcn1/1 -> Real-Imag to Complex/2  "beta"
  Fcn/1 -> Real-Imag to Complex/1  "alpha"
  vs_abc/1 -> Fcn/1, Fcn1/1

== system JONASBROTHERS/Indirect Field oriented control/IM/alphabeta->abc ==
  note: u(2)
  note: u(1)
  note: u(2)
  note: u(1)
  note: u(2)
  note: u(1)
  i_s^s : Inport
  Complex to Real-Imag : ComplexToRealImag
  Fcn : Fcn  Expr=u(1)
  Fcn1 : Fcn  Expr=-0.5*u(1)+0.5*sqrt(3)*u(2)
  Fcn2 : Fcn  Expr=-0.5*u(1)-0.5*sqrt(3)*u(2)
  Mux : Mux  Inputs=2
  Mux1 : Mux  Inputs=2
  Mux2 : Mux  Inputs=2
  Mux3 : Mux  Inputs=3
  is_abc : Outport
  wires:
  Mux3/1 -> is_abc/1
  Fcn2/1 -> Mux3/3
  Fcn1/1 -> Mux3/2
  Fcn/1 -> Mux3/1
  i_s^s/1 -> Complex to Real-Imag/1
  Mux2/1 -> Fcn2/1
  Mux1/1 -> Fcn1/1
  Complex to Real-Imag/2 -> Mux2/2, Mux1/2, Mux/2  "beta"
  Complex to Real-Imag/1 -> Mux2/1, Mux1/1, Mux/1  "alpha"
  Mux/1 -> Fcn/1

== system JONASBROTHERS/Indirect Field oriented control/IM/Voltage Equations/Integrator (Complex Signal) ==
  u : Inport
  Complex to Real-Imag : ComplexToRealImag
  Integrator : Integrator  InitialCondition=psi_ref
  Integrator1 : Integrator
  Real-Imag to Complex : RealImagToComplex
  y : Outport
  wires:
  u/1 -> Complex to Real-Imag/1
  Real-Imag to Complex/1 -> y/1
  Integrator1/1 -> Real-Imag to Complex/2
  Integrator/1 -> Real-Imag to Complex/1
  Complex to Real-Imag/2 -> Integrator1/1
  Complex to Real-Imag/1 -> Integrator/1

== system JONASBROTHERS/Indirect Field oriented control/IM/Voltage Equations/Integrator (Complex Signal)1 ==
  u : Inport
  Complex to Real-Imag : ComplexToRealImag
  Integrator : Integrator  InitialCondition=psi_ref
  Integrator1 : Integrator
  Real-Imag to Complex : RealImagToComplex
  y : Outport
  wires:
  u/1 -> Complex to Real-Imag/1
  Real-Imag to Complex/1 -> y/1
  Integrator1/1 -> Real-Imag to Complex/2
  Integrator/1 -> Real-Imag to Complex/1
  Complex to Real-Imag/2 -> Integrator1/1
  Complex to Real-Imag/1 -> Integrator/1
